simulink model "Ejercicio17_20_02_17"  (R2013a)
settings: Solver=ode45  StartTime=0.0  StopTime=100  RelTol=1e-3
settings Model: Creator=Miguel  LastModifiedBy=Miguel

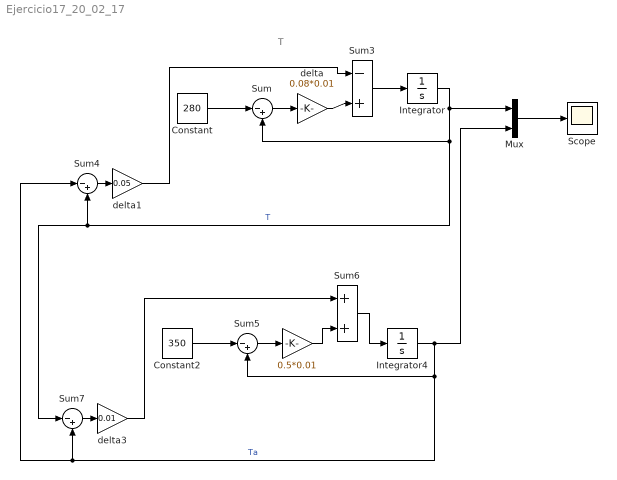
== system Ejercicio17_20_02_17 ==
  note: T
  " " : Gain  Gain=0.5*0.01
  Constant : Constant  Value=280
  Constant2 : Constant  Value=350
  Integrator : Integrator  InitialCondition=280
  Integrator4 : Integrator  InitialCondition=350
  Mux : Mux  Inputs=2
  Scope : Scope
      settings: ShowLegends=on  TimeRange=10
  Sum{,3..5,7} (5 alike) : Sum  Inputs=|-+
  Sum6 : Sum  Inputs=|++
  delta : Gain  Gain=0.08*0.01
  delta1 : Gain  Gain=0.05
  delta3 : Gain  Gain=0.01
  wires:
  Sum/1 -> delta/1
  Mux/1 -> Scope/1
  Constant/1 -> Sum/1
  delta/1 -> Sum3/2
  Sum4/1 -> delta1/1
  Integrator/1 -> Mux/1, Sum7/1, Sum4/2, Sum/2  "T"
  delta1/1 -> Sum3/1
  Sum5/1 -> " "/1
  Constant2/1 -> Sum5/1
  " "/1 -> Sum6/2
  Sum7/1 -> delta3/1
  Integrator4/1 -> Mux/2, Sum4/1, Sum7/2, Sum5/2  "Ta"
  delta3/1 -> Sum6/1
  Sum6/1 -> Integrator4/1
  Sum3/1 -> Integrator/1
